simulink model "gm_parallel_lht"  (R2019b)
settings: Solver=FixedStepDiscrete  StartTime=0.0  StopTime=inf  RelTol=1e-3
undefined symbols (not defined in the file or in its folder): bt, height, width
libraries: hdlsllib x190, simulink x13, hdlmdlgenlib x7, dspsrcs4 x1
(part 2 of 18)

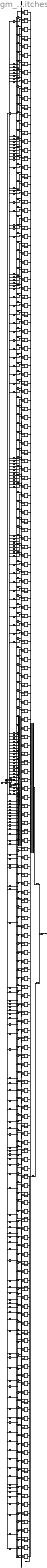
== system gm_parallel_lht/Parallel LHT/Parallel LHT Accumulator/Accumulator with Switches ==
  hough_address : Inport  OutDataTypeStr=fixdt(0, 11, 0)  PortDimensions=[1 180]  SampleTime=6.66666666666667e-09
  edge : Inport  Port=2  OutDataTypeStr=boolean  PortDimensions=1  SampleTime=6.66666666666667e-09
  mode : Inport  Port=3  OutDataTypeStr=boolean  PortDimensions=1  SampleTime=6.66666666666667e-09
  read_address : Inport  Port=4  OutDataTypeStr=uint16  PortDimensions=1  SampleTime=6.66666666666667e-09
  clear : Inport  Port=5  OutDataTypeStr=boolean  PortDimensions=1  SampleTime=6.66666666666667e-09
  theta_index : Inport  Port=6  OutDataTypeStr=uint16  PortDimensions=1  SampleTime=6.66666666666667e-09
  Accumulator_instance1 : Subsystem
  Accumulator_instance10 : Subsystem
  Accumulator_instance100 : Subsystem
  Accumulator_instance101 : Subsystem
  Accumulator_instance102 : Subsystem
  Accumulator_instance103 : Subsystem
  Accumulator_instance104 : Subsystem
  Accumulator_instance105 : Subsystem
  Accumulator_instance106 : Subsystem
  Accumulator_instance107 : Subsystem
  Accumulator_instance108 : Subsystem
  Accumulator_instance109 : Subsystem
  Accumulator_instance11 : Subsystem
  Accumulator_instance110 : Subsystem
  Accumulator_instance111 : Subsystem
  Accumulator_instance112 : Subsystem
  Accumulator_instance113 : Subsystem
  Accumulator_instance114 : Subsystem
  Accumulator_instance115 : Subsystem
  Accumulator_instance116 : Subsystem
  Accumulator_instance117 : Subsystem
  Accumulator_instance118 : Subsystem
  Accumulator_instance119 : Subsystem
  Accumulator_instance12 : Subsystem
  Accumulator_instance120 : Subsystem
  Accumulator_instance121 : Subsystem
  Accumulator_instance122 : Subsystem
  Accumulator_instance123 : Subsystem
  Accumulator_instance124 : Subsystem
  Accumulator_instance125 : Subsystem
  Accumulator_instance126 : Subsystem
  Accumulator_instance127 : Subsystem
  Accumulator_instance128 : Subsystem
  Accumulator_instance129 : Subsystem
  Accumulator_instance13 : Subsystem
  Accumulator_instance130 : Subsystem
  Accumulator_instance131 : Subsystem
  Accumulator_instance132 : Subsystem
  Accumulator_instance133 : Subsystem
  Accumulator_instance134 : Subsystem
  Accumulator_instance135 : Subsystem
  Accumulator_instance136 : Subsystem
  Accumulator_instance137 : Subsystem
  Accumulator_instance138 : Subsystem
  Accumulator_instance139 : Subsystem
  Accumulator_instance14 : Subsystem
  Accumulator_instance140 : Subsystem
  Accumulator_instance141 : Subsystem
  Accumulator_instance142 : Subsystem
  Accumulator_instance143 : Subsystem
  Accumulator_instance144 : Subsystem
  Accumulator_instance145 : Subsystem
  Accumulator_instance146 : Subsystem
  Accumulator_instance147 : Subsystem
  Accumulator_instance148 : Subsystem
  Accumulator_instance149 : Subsystem
  Accumulator_instance15 : Subsystem
  Accumulator_instance150 : Subsystem
  Accumulator_instance151 : Subsystem
  Accumulator_instance152 : Subsystem
  Accumulator_instance153 : Subsystem
  Accumulator_instance154 : Subsystem
  Accumulator_instance155 : Subsystem
  Accumulator_instance156 : Subsystem
  Accumulator_instance157 : Subsystem
  Accumulator_instance158 : Subsystem
  Accumulator_instance159 : Subsystem
  Accumulator_instance16 : Subsystem
  Accumulator_instance160 : Subsystem
  Accumulator_instance161 : Subsystem
  Accumulator_instance162 : Subsystem
  Accumulator_instance163 : Subsystem
  Accumulator_instance164 : Subsystem
  Accumulator_instance165 : Subsystem
  Accumulator_instance166 : Subsystem
  Accumulator_instance167 : Subsystem
  Accumulator_instance168 : Subsystem
  Accumulator_instance169 : Subsystem
  Accumulator_instance17 : Subsystem
  Accumulator_instance170 : Subsystem
  Accumulator_instance171 : Subsystem
  Accumulator_instance172 : Subsystem
  Accumulator_instance173 : Subsystem
  Accumulator_instance174 : Subsystem
  Accumulator_instance175 : Subsystem
  Accumulator_instance176 : Subsystem
  Accumulator_instance177 : Subsystem
  Accumulator_instance178 : Subsystem
  Accumulator_instance179 : Subsystem
  Accumulator_instance18 : Subsystem
  Accumulator_instance180 : Subsystem
  Accumulator_instance19 : Subsystem
  Accumulator_instance2 : Subsystem
  Accumulator_instance20 : Subsystem
  Accumulator_instance21 : Subsystem
  Accumulator_instance22 : Subsystem
  Accumulator_instance23 : Subsystem
  Accumulator_instance24 : Subsystem
  Accumulator_instance25 : Subsystem
  Accumulator_instance26 : Subsystem
  Accumulator_instance27 : Subsystem
  Accumulator_instance28 : Subsystem
  Accumulator_instance29 : Subsystem
  Accumulator_instance3 : Subsystem
  Accumulator_instance30 : Subsystem
  Accumulator_instance31 : Subsystem
  Accumulator_instance32 : Subsystem
  Accumulator_instance33 : Subsystem
  Accumulator_instance34 : Subsystem
  Accumulator_instance35 : Subsystem
  Accumulator_instance36 : Subsystem
  Accumulator_instance37 : Subsystem
  Accumulator_instance38 : Subsystem
  Accumulator_instance39 : Subsystem
  Accumulator_instance4 : Subsystem
  Accumulator_instance40 : Subsystem
  Accumulator_instance41 : Subsystem
  Accumulator_instance42 : Subsystem
  Accumulator_instance43 : Subsystem
  Accumulator_instance44 : Subsystem
  Accumulator_instance45 : Subsystem
  Accumulator_instance46 : Subsystem
  Accumulator_instance47 : Subsystem
  Accumulator_instance48 : Subsystem
  Accumulator_instance49 : Subsystem
  Accumulator_instance5 : Subsystem
  Accumulator_instance50 : Subsystem
  Accumulator_instance51 : Subsystem
  Accumulator_instance52 : Subsystem
  Accumulator_instance53 : Subsystem
  Accumulator_instance54 : Subsystem
  Accumulator_instance55 : Subsystem
  Accumulator_instance56 : Subsystem
  Accumulator_instance57 : Subsystem
  Accumulator_instance58 : Subsystem
  Accumulator_instance59 : Subsystem
  Accumulator_instance6 : Subsystem
  Accumulator_instance60 : Subsystem
  Accumulator_instance61 : Subsystem
  Accumulator_instance62 : Subsystem
  Accumulator_instance63 : Subsystem
  Accumulator_instance64 : Subsystem
  Accumulator_instance65 : Subsystem
  Accumulator_instance66 : Subsystem
  Accumulator_instance67 : Subsystem
  Accumulator_instance68 : Subsystem
  Accumulator_instance69 : Subsystem
  Accumulator_instance7 : Subsystem
  Accumulator_instance70 : Subsystem
  Accumulator_instance71 : Subsystem
  Accumulator_instance72 : Subsystem
  Accumulator_instance73 : Subsystem
  Accumulator_instance74 : Subsystem
  Accumulator_instance75 : Subsystem
  Accumulator_instance76 : Subsystem
  Accumulator_instance77 : Subsystem
  Accumulator_instance78 : Subsystem
  Accumulator_instance79 : Subsystem
  Accumulator_instance8 : Subsystem
  Accumulator_instance80 : Subsystem
  Accumulator_instance81 : Subsystem
  Accumulator_instance82 : Subsystem
  Accumulator_instance83 : Subsystem
  Accumulator_instance84 : Subsystem
  Accumulator_instance85 : Subsystem
  Accumulator_instance86 : Subsystem
  Accumulator_instance87 : Subsystem
  Accumulator_instance88 : Subsystem
  Accumulator_instance89 : Subsystem
  Accumulator_instance9 : Subsystem
  Accumulator_instance90 : Subsystem
  Accumulator_instance91 : Subsystem
  Accumulator_instance92 : Subsystem
  Accumulator_instance93 : Subsystem
  Accumulator_instance94 : Subsystem
  Accumulator_instance95 : Subsystem
  Accumulator_instance96 : Subsystem
  Accumulator_instance97 : Subsystem
  Accumulator_instance98 : Subsystem
  Accumulator_instance99 : Subsystem
  Data Type Conversion : DataTypeConversion  OutDataTypeStr=fixdt(0, 11, 0)  SampleTime=6.66666666666667e-09
  Delay : Delay  DelayLength=double(1)  InitialCondition=0  SampleTime=6.66666666666667e-09
  Multiport Switch1 : MultiPortSwitch  DataPortOrder=Zero-based contiguous  Inputs=2  DiagnosticForDefault=None  zeroidx=on  SampleTime=6.66666666666667e-09
  Selector : Selector  NumberOfDimensions=2  IndexMode=Zero-based  SampleTime=6.66666666666667e-09  IndexOptions=Index vector (dialog),Index vector (port)  Indices=double(0),double(0)  OutputSizes=double(1),double(1)
  Switch : Switch  Criteria=u2 > Threshold  Threshold=double(0)  OutDataTypeStr=fixdt(0, 11, 0)  SampleTime=6.66666666666667e-09
  delayMatch{,1..362} (363 alike) : Delay  DelayLength=double(2)  InitialCondition=0  SampleTime=6.66666666666667e-09
  t : Demux  Outputs=180
  t1 : Concatenate  NumInputs=180
  t2 : Reshape  OutputDimensionality=Row vector (2-D)
  hps : Outport
  wires:
  delayMatch/1 -> Switch/2
  t2/1 -> Selector/1
  delayMatch1/1 -> Switch/3
  delayMatch362/1 -> Selector/2
  delayMatch3/1 -> Accumulator_instance1/3(edge)
  Selector/1 -> hps/1
  Switch/1 -> t/1
  t/1 -> Accumulator_instance1/2(address)
  t/2 -> Accumulator_instance2/2(address)
  t/3 -> Accumulator_instance3/2(address)
  t/4 -> Accumulator_instance4/2(address)
  t/5 -> Accumulator_instance5/2(address)
  t/6 -> Accumulator_instance6/2(address)
  t/7 -> Accumulator_instance7/2(address)
  t/8 -> Accumulator_instance8/2(address)
  t/9 -> Accumulator_instance9/2(address)
  t/10 -> Accumulator_instance10/2(address)
  t/11 -> Accumulator_instance11/2(address)
  t/12 -> Accumulator_instance12/2(address)
  t/13 -> Accumulator_instance13/2(address)
  t/14 -> Accumulator_instance14/2(address)
  t/15 -> Accumulator_instance15/2(address)
  t/16 -> Accumulator_instance16/2(address)
  t/17 -> Accumulator_instance17/2(address)
  t/18 -> Accumulator_instance18/2(address)
  t/19 -> Accumulator_instance19/2(address)
  t/20 -> Accumulator_instance20/2(address)
  t/21 -> Accumulator_instance21/2(address)
  t/22 -> Accumulator_instance22/2(address)
  t/23 -> Accumulator_instance23/2(address)
  t/24 -> Accumulator_instance24/2(address)
  t/25 -> Accumulator_instance25/2(address)
  t/26 -> Accumulator_instance26/2(address)
  t/27 -> Accumulator_instance27/2(address)
  t/28 -> Accumulator_instance28/2(address)
  t/29 -> Accumulator_instance29/2(address)
  t/30 -> Accumulator_instance30/2(address)
  t/31 -> Accumulator_instance31/2(address)
  t/32 -> Accumulator_instance32/2(address)
  t/33 -> Accumulator_instance33/2(address)
  t/34 -> Accumulator_instance34/2(address)
  t/35 -> Accumulator_instance35/2(address)
  t/36 -> Accumulator_instance36/2(address)
  t/37 -> Accumulator_instance37/2(address)
  t/38 -> Accumulator_instance38/2(address)
  t/39 -> Accumulator_instance39/2(address)
  t/40 -> Accumulator_instance40/2(address)
  t/41 -> Accumulator_instance41/2(address)
  t/42 -> Accumulator_instance42/2(address)
  t/43 -> Accumulator_instance43/2(address)
  t/44 -> Accumulator_instance44/2(address)
  t/45 -> Accumulator_instance45/2(address)
  t/46 -> Accumulator_instance46/2(address)
  t/47 -> Accumulator_instance47/2(address)
  t/48 -> Accumulator_instance48/2(address)
  t/49 -> Accumulator_instance49/2(address)
  t/50 -> Accumulator_instance50/2(address)
  t/51 -> Accumulator_instance51/2(address)
  t/52 -> Accumulator_instance52/2(address)
  t/53 -> Accumulator_instance53/2(address)
  t/54 -> Accumulator_instance54/2(address)
  t/55 -> Accumulator_instance55/2(address)
  t/56 -> Accumulator_instance56/2(address)
  t/57 -> Accumulator_instance57/2(address)
  t/58 -> Accumulator_instance58/2(address)
  t/59 -> Accumulator_instance59/2(address)
  t/60 -> Accumulator_instance60/2(address)
  t/61 -> Accumulator_instance61/2(address)
  t/62 -> Accumulator_instance62/2(address)
  t/63 -> Accumulator_instance63/2(address)
  t/64 -> Accumulator_instance64/2(address)
  t/65 -> Accumulator_instance65/2(address)
  t/66 -> Accumulator_instance66/2(address)
  t/67 -> Accumulator_instance67/2(address)
  t/68 -> Accumulator_instance68/2(address)
  t/69 -> Accumulator_instance69/2(address)
  t/70 -> Accumulator_instance70/2(address)
  t/71 -> Accumulator_instance71/2(address)
  t/72 -> Accumulator_instance72/2(address)
  t/73 -> Accumulator_instance73/2(address)
  t/74 -> Accumulator_instance74/2(address)
  t/75 -> Accumulator_instance75/2(address)
  t/76 -> Accumulator_instance76/2(address)
  t/77 -> Accumulator_instance77/2(address)
  t/78 -> Accumulator_instance78/2(address)
  t/79 -> Accumulator_instance79/2(address)
  t/80 -> Accumulator_instance80/2(address)
  t/81 -> Accumulator_instance81/2(address)
  t/82 -> Accumulator_instance82/2(address)
  t/83 -> Accumulator_instance83/2(address)
  t/84 -> Accumulator_instance84/2(address)
  t/85 -> Accumulator_instance85/2(address)
  t/86 -> Accumulator_instance86/2(address)
  t/87 -> Accumulator_instance87/2(address)
  t/88 -> Accumulator_instance88/2(address)
  t/89 -> Accumulator_instance89/2(address)
  t/90 -> Accumulator_instance90/2(address)
  t/91 -> Accumulator_instance91/2(address)
  t/92 -> Accumulator_instance92/2(address)
  t/93 -> Accumulator_instance93/2(address)
  t/94 -> Accumulator_instance94/2(address)
  t/95 -> Accumulator_instance95/2(address)
  t/96 -> Accumulator_instance96/2(address)
  t/97 -> Accumulator_instance97/2(address)
  t/98 -> Accumulator_instance98/2(address)
  t/99 -> Accumulator_instance99/2(address)
  t/100 -> Accumulator_instance100/2(address)
  t/101 -> Accumulator_instance101/2(address)
  t/102 -> Accumulator_instance102/2(address)
  t/103 -> Accumulator_instance103/2(address)
  t/104 -> Accumulator_instance104/2(address)
  t/105 -> Accumulator_instance105/2(address)
  t/106 -> Accumulator_instance106/2(address)
  t/107 -> Accumulator_instance107/2(address)
  t/108 -> Accumulator_instance108/2(address)
  t/109 -> Accumulator_instance109/2(address)
  t/110 -> Accumulator_instance110/2(address)
  t/111 -> Accumulator_instance111/2(address)
  t/112 -> Accumulator_instance112/2(address)
  t/113 -> Accumulator_instance113/2(address)
  t/114 -> Accumulator_instance114/2(address)
  t/115 -> Accumulator_instance115/2(address)
  t/116 -> Accumulator_instance116/2(address)
  t/117 -> Accumulator_instance117/2(address)
  t/118 -> Accumulator_instance118/2(address)
  t/119 -> Accumulator_instance119/2(address)
  t/120 -> Accumulator_instance120/2(address)
  t/121 -> Accumulator_instance121/2(address)
  t/122 -> Accumulator_instance122/2(address)
  t/123 -> Accumulator_instance123/2(address)
  t/124 -> Accumulator_instance124/2(address)
  t/125 -> Accumulator_instance125/2(address)
  t/126 -> Accumulator_instance126/2(address)
  t/127 -> Accumulator_instance127/2(address)
  t/128 -> Accumulator_instance128/2(address)
  t/129 -> Accumulator_instance129/2(address)
  t/130 -> Accumulator_instance130/2(address)
  t/131 -> Accumulator_instance131/2(address)
  t/132 -> Accumulator_instance132/2(address)
  t/133 -> Accumulator_instance133/2(address)
  t/134 -> Accumulator_instance134/2(address)
  t/135 -> Accumulator_instance135/2(address)
  t/136 -> Accumulator_instance136/2(address)
  t/137 -> Accumulator_instance137/2(address)
  t/138 -> Accumulator_instance138/2(address)
  t/139 -> Accumulator_instance139/2(address)
  t/140 -> Accumulator_instance140/2(address)
  t/141 -> Accumulator_instance141/2(address)
  t/142 -> Accumulator_instance142/2(address)
  t/143 -> Accumulator_instance143/2(address)
  t/144 -> Accumulator_instance144/2(address)
  t/145 -> Accumulator_instance145/2(address)
  t/146 -> Accumulator_instance146/2(address)
  t/147 -> Accumulator_instance147/2(address)
  t/148 -> Accumulator_instance148/2(address)
  t/149 -> Accumulator_instance149/2(address)
  t/150 -> Accumulator_instance150/2(address)
  t/151 -> Accumulator_instance151/2(address)
  t/152 -> Accumulator_instance152/2(address)
  t/153 -> Accumulator_instance153/2(address)
  t/154 -> Accumulator_instance154/2(address)
  t/155 -> Accumulator_instance155/2(address)
  t/156 -> Accumulator_instance156/2(address)
  t/157 -> Accumulator_instance157/2(address)
  t/158 -> Accumulator_instance158/2(address)
  t/159 -> Accumulator_instance159/2(address)
  t/160 -> Accumulator_instance160/2(address)
  t/161 -> Accumulator_instance161/2(address)
  t/162 -> Accumulator_instance162/2(address)
  t/163 -> Accumulator_instance163/2(address)
  t/164 -> Accumulator_instance164/2(address)
  t/165 -> Accumulator_instance165/2(address)
  t/166 -> Accumulator_instance166/2(address)
  t/167 -> Accumulator_instance167/2(address)
  t/168 -> Accumulator_instance168/2(address)
  t/169 -> Accumulator_instance169/2(address)
  t/170 -> Accumulator_instance170/2(address)
  t/171 -> Accumulator_instance171/2(address)
  t/172 -> Accumulator_instance172/2(address)
  t/173 -> Accumulator_instance173/2(address)
  t/174 -> Accumulator_instance174/2(address)
  t/175 -> Accumulator_instance175/2(address)
  t/176 -> Accumulator_instance176/2(address)
  t/177 -> Accumulator_instance177/2(address)
  t/178 -> Accumulator_instance178/2(address)
  t/179 -> Accumulator_instance179/2(address)
  t/180 -> Accumulator_instance180/2(address)
  t1/1 -> t2/1
  Accumulator_instance1/1(hps) -> t1/1
  Accumulator_instance2/1(hps) -> t1/2
  Accumulator_instance3/1(hps) -> t1/3
  Accumulator_instance4/1(hps) -> t1/4
  Accumulator_instance5/1(hps) -> t1/5
  Accumulator_instance6/1(hps) -> t1/6
  Accumulator_instance7/1(hps) -> t1/7
  Accumulator_instance8/1(hps) -> t1/8
  Accumulator_instance9/1(hps) -> t1/9
  Accumulator_instance10/1(hps) -> t1/10
  Accumulator_instance11/1(hps) -> t1/11
  Accumulator_instance12/1(hps) -> t1/12
  Accumulator_instance13/1(hps) -> t1/13
  Accumulator_instance14/1(hps) -> t1/14
  Accumulator_instance15/1(hps) -> t1/15
  Accumulator_instance16/1(hps) -> t1/16
  Accumulator_instance17/1(hps) -> t1/17
  Accumulator_instance18/1(hps) -> t1/18
  Accumulator_instance19/1(hps) -> t1/19
  Accumulator_instance20/1(hps) -> t1/20
  Accumulator_instance21/1(hps) -> t1/21
  Accumulator_instance22/1(hps) -> t1/22
  Accumulator_instance23/1(hps) -> t1/23
  Accumulator_instance24/1(hps) -> t1/24
  Accumulator_instance25/1(hps) -> t1/25
  Accumulator_instance26/1(hps) -> t1/26
  Accumulator_instance27/1(hps) -> t1/27
  Accumulator_instance28/1(hps) -> t1/28
  Accumulator_instance29/1(hps) -> t1/29
  Accumulator_instance30/1(hps) -> t1/30
  Accumulator_instance31/1(hps) -> t1/31
  Accumulator_instance32/1(hps) -> t1/32
  Accumulator_instance33/1(hps) -> t1/33
  Accumulator_instance34/1(hps) -> t1/34
  Accumulator_instance35/1(hps) -> t1/35
  Accumulator_instance36/1(hps) -> t1/36
  Accumulator_instance37/1(hps) -> t1/37
  Accumulator_instance38/1(hps) -> t1/38
  Accumulator_instance39/1(hps) -> t1/39
  Accumulator_instance40/1(hps) -> t1/40
  Accumulator_instance41/1(hps) -> t1/41
  Accumulator_instance42/1(hps) -> t1/42
  Accumulator_instance43/1(hps) -> t1/43
  Accumulator_instance44/1(hps) -> t1/44
  Accumulator_instance45/1(hps) -> t1/45
  Accumulator_instance46/1(hps) -> t1/46
  Accumulator_instance47/1(hps) -> t1/47
  Accumulator_instance48/1(hps) -> t1/48
  Accumulator_instance49/1(hps) -> t1/49
  Accumulator_instance50/1(hps) -> t1/50
  Accumulator_instance51/1(hps) -> t1/51
  Accumulator_instance52/1(hps) -> t1/52
  Accumulator_instance53/1(hps) -> t1/53
  Accumulator_instance54/1(hps) -> t1/54
  Accumulator_instance55/1(hps) -> t1/55
  Accumulator_instance56/1(hps) -> t1/56
  Accumulator_instance57/1(hps) -> t1/57
  Accumulator_instance58/1(hps) -> t1/58
  Accumulator_instance59/1(hps) -> t1/59
  Accumulator_instance60/1(hps) -> t1/60
  Accumulator_instance61/1(hps) -> t1/61
  Accumulator_instance62/1(hps) -> t1/62
  Accumulator_instance63/1(hps) -> t1/63
  Accumulator_instance64/1(hps) -> t1/64
  Accumulator_instance65/1(hps) -> t1/65
  Accumulator_instance66/1(hps) -> t1/66
  Accumulator_instance67/1(hps) -> t1/67
  Accumulator_instance68/1(hps) -> t1/68
  Accumulator_instance69/1(hps) -> t1/69
  Accumulator_instance70/1(hps) -> t1/70
  Accumulator_instance71/1(hps) -> t1/71
  Accumulator_instance72/1(hps) -> t1/72
  Accumulator_instance73/1(hps) -> t1/73
  Accumulator_instance74/1(hps) -> t1/74
  Accumulator_instance75/1(hps) -> t1/75
  Accumulator_instance76/1(hps) -> t1/76
  Accumulator_instance77/1(hps) -> t1/77
  Accumulator_instance78/1(hps) -> t1/78
  Accumulator_instance79/1(hps) -> t1/79
  Accumulator_instance80/1(hps) -> t1/80
  Accumulator_instance81/1(hps) -> t1/81
  Accumulator_instance82/1(hps) -> t1/82
  Accumulator_instance83/1(hps) -> t1/83
  Accumulator_instance84/1(hps) -> t1/84
  Accumulator_instance85/1(hps) -> t1/85
  Accumulator_instance86/1(hps) -> t1/86
  Accumulator_instance87/1(hps) -> t1/87
  Accumulator_instance88/1(hps) -> t1/88
  Accumulator_instance89/1(hps) -> t1/89
  Accumulator_instance90/1(hps) -> t1/90
  Accumulator_instance91/1(hps) -> t1/91
  Accumulator_instance92/1(hps) -> t1/92
  Accumulator_instance93/1(hps) -> t1/93
  Accumulator_instance94/1(hps) -> t1/94
  Accumulator_instance95/1(hps) -> t1/95
  Accumulator_instance96/1(hps) -> t1/96
  Accumulator_instance97/1(hps) -> t1/97
  Accumulator_instance98/1(hps) -> t1/98
  Accumulator_instance99/1(hps) -> t1/99
  Accumulator_instance100/1(hps) -> t1/100
  Accumulator_instance101/1(hps) -> t1/101
  Accumulator_instance102/1(hps) -> t1/102
  Accumulator_instance103/1(hps) -> t1/103
  Accumulator_instance104/1(hps) -> t1/104
  Accumulator_instance105/1(hps) -> t1/105
  Accumulator_instance106/1(hps) -> t1/106
  Accumulator_instance107/1(hps) -> t1/107
  Accumulator_instance108/1(hps) -> t1/108
  Accumulator_instance109/1(hps) -> t1/109
  Accumulator_instance110/1(hps) -> t1/110
  Accumulator_instance111/1(hps) -> t1/111
  Accumulator_instance112/1(hps) -> t1/112
  Accumulator_instance113/1(hps) -> t1/113
  Accumulator_instance114/1(hps) -> t1/114
  Accumulator_instance115/1(hps) -> t1/115
  Accumulator_instance116/1(hps) -> t1/116
  Accumulator_instance117/1(hps) -> t1/117
  Accumulator_instance118/1(hps) -> t1/118
  Accumulator_instance119/1(hps) -> t1/119
  Accumulator_instance120/1(hps) -> t1/120
  Accumulator_instance121/1(hps) -> t1/121
  Accumulator_instance122/1(hps) -> t1/122
  Accumulator_instance123/1(hps) -> t1/123
  Accumulator_instance124/1(hps) -> t1/124
  Accumulator_instance125/1(hps) -> t1/125
  Accumulator_instance126/1(hps) -> t1/126
  Accumulator_instance127/1(hps) -> t1/127
  Accumulator_instance128/1(hps) -> t1/128
  Accumulator_instance129/1(hps) -> t1/129
  Accumulator_instance130/1(hps) -> t1/130
  Accumulator_instance131/1(hps) -> t1/131
  Accumulator_instance132/1(hps) -> t1/132
  Accumulator_instance133/1(hps) -> t1/133
  Accumulator_instance134/1(hps) -> t1/134
  Accumulator_instance135/1(hps) -> t1/135
  Accumulator_instance136/1(hps) -> t1/136
  Accumulator_instance137/1(hps) -> t1/137
  Accumulator_instance138/1(hps) -> t1/138
  Accumulator_instance139/1(hps) -> t1/139
  Accumulator_instance140/1(hps) -> t1/140
  Accumulator_instance141/1(hps) -> t1/141
  Accumulator_instance142/1(hps) -> t1/142
  Accumulator_instance143/1(hps) -> t1/143
  Accumulator_instance144/1(hps) -> t1/144
  Accumulator_instance145/1(hps) -> t1/145
  Accumulator_instance146/1(hps) -> t1/146
  Accumulator_instance147/1(hps) -> t1/147
  Accumulator_instance148/1(hps) -> t1/148
  Accumulator_instance149/1(hps) -> t1/149
  Accumulator_instance150/1(hps) -> t1/150
  Accumulator_instance151/1(hps) -> t1/151
  Accumulator_instance152/1(hps) -> t1/152
  Accumulator_instance153/1(hps) -> t1/153
  Accumulator_instance154/1(hps) -> t1/154
  Accumulator_instance155/1(hps) -> t1/155
  Accumulator_instance156/1(hps) -> t1/156
  Accumulator_instance157/1(hps) -> t1/157
  Accumulator_instance158/1(hps) -> t1/158
  Accumulator_instance159/1(hps) -> t1/159
  Accumulator_instance160/1(hps) -> t1/160
  Accumulator_instance161/1(hps) -> t1/161
  Accumulator_instance162/1(hps) -> t1/162
  Accumulator_instance163/1(hps) -> t1/163
  Accumulator_instance164/1(hps) -> t1/164
  Accumulator_instance165/1(hps) -> t1/165
  Accumulator_instance166/1(hps) -> t1/166
  Accumulator_instance167/1(hps) -> t1/167
  Accumulator_instance168/1(hps) -> t1/168
  Accumulator_instance169/1(hps) -> t1/169
  Accumulator_instance170/1(hps) -> t1/170
  Accumulator_instance171/1(hps) -> t1/171
  Accumulator_instance172/1(hps) -> t1/172
  Accumulator_instance173/1(hps) -> t1/173
  Accumulator_instance174/1(hps) -> t1/174
  Accumulator_instance175/1(hps) -> t1/175
  Accumulator_instance176/1(hps) -> t1/176
  Accumulator_instance177/1(hps) -> t1/177
  Accumulator_instance178/1(hps) -> t1/178
  Accumulator_instance179/1(hps) -> t1/179
  Accumulator_instance180/1(hps) -> t1/180
  hough_address/1 -> Switch/1
  edge/1 -> Multiport Switch1/3
  mode/1 -> delayMatch360/1, delayMatch358/1, delayMatch356/1, delayMatch354/1, delayMatch352/1, delayMatch350/1, delayMatch348/1, delayMatch346/1, delayMatch344/1, delayMatch342/1, delayMatch340/1, delayMatch338/1, delayMatch336/1, delayMatch334/1, delayMatch332/1, delayMatch330/1, delayMatch328/1, delayMatch326/1, delayMatch324/1, delayMatch322/1, delayMatch320/1, delayMatch318/1, delayMatch316/1, delayMatch314/1, delayMatch312/1, delayMatch310/1, delayMatch308/1, delayMatch306/1, delayMatch304/1, delayMatch302/1, delayMatch300/1, delayMatch298/1, delayMatch296/1, delayMatch294/1, delayMatch292/1, delayMatch290/1, delayMatch288/1, delayMatch286/1, delayMatch284/1, delayMatch282/1, delayMatch280/1, delayMatch278/1, delayMatch276/1, delayMatch274/1, delayMatch272/1, delayMatch270/1, delayMatch268/1, delayMatch266/1, delayMatch264/1, delayMatch262/1, delayMatch260/1, delayMatch258/1, delayMatch256/1, delayMatch254/1, delayMatch252/1, delayMatch250/1, delayMatch248/1, delayMatch246/1, delayMatch244/1, delayMatch242/1, delayMatch240/1, delayMatch238/1, delayMatch236/1, delayMatch234/1, delayMatch232/1, delayMatch230/1, delayMatch228/1, delayMatch226/1, delayMatch224/1, delayMatch222/1, delayMatch220/1, delayMatch218/1, delayMatch216/1, delayMatch214/1, delayMatch212/1, delayMatch210/1, delayMatch208/1, delayMatch206/1, delayMatch204/1, delayMatch202/1, delayMatch200/1, delayMatch198/1, delayMatch196/1, delayMatch194/1, delayMatch192/1, delayMatch190/1, delayMatch188/1, delayMatch186/1, delayMatch184/1, delayMatch182/1, delayMatch180/1, delayMatch178/1, delayMatch176/1, delayMatch174/1, delayMatch172/1, delayMatch170/1, delayMatch168/1, delayMatch166/1, delayMatch164/1, delayMatch162/1, delayMatch160/1, delayMatch158/1, delayMatch156/1, delayMatch154/1, delayMatch152/1, delayMatch150/1, delayMatch148/1, delayMatch146/1, delayMatch144/1, delayMatch142/1, delayMatch140/1, delayMatch138/1, delayMatch136/1, delayMatch134/1, delayMatch132/1, delayMatch130/1, delayMatch128/1, delayMatch126/1, delayMatch124/1, delayMatch122/1, delayMatch120/1, delayMatch118/1, delayMatch116/1, delayMatch114/1, delayMatch112/1, delayMatch110/1, delayMatch108/1, delayMatch106/1, delayMatch104/1, delayMatch102/1, delayMatch100/1, delayMatch98/1, delayMatch96/1, delayMatch94/1, delayMatch92/1, delayMatch90/1, delayMatch88/1, delayMatch86/1, delayMatch84/1, delayMatch82/1, delayMatch80/1, delayMatch78/1, delayMatch76/1, delayMatch74/1, delayMatch72/1, delayMatch70/1, delayMatch68/1, delayMatch66/1, delayMatch64/1, delayMatch62/1, delayMatch60/1, delayMatch58/1, delayMatch56/1, delayMatch54/1, delayMatch52/1, delayMatch50/1, delayMatch48/1, delayMatch46/1, delayMatch44/1, delayMatch42/1, delayMatch40/1, delayMatch38/1, delayMatch36/1, delayMatch34/1, delayMatch32/1, delayMatch30/1, delayMatch28/1, delayMatch26/1, delayMatch24/1, delayMatch22/1, delayMatch20/1, delayMatch18/1, delayMatch16/1, delayMatch14/1, delayMatch12/1, delayMatch10/1, delayMatch8/1, delayMatch6/1, delayMatch4/1, delayMatch2/1, delayMatch/1, Multiport Switch1/1
  read_address/1 -> Data Type Conversion/1
  clear/1 -> Multiport Switch1/2
  theta_index/1 -> Delay/1
  delayMatch2/1 -> Accumulator_instance1/1(mode)
  Data Type Conversion/1 -> delayMatch1/1
  delayMatch4/1 -> Accumulator_instance2/1(mode)
  delayMatch5/1 -> Accumulator_instance2/3(edge)
  delayMatch6/1 -> Accumulator_instance3/1(mode)
  delayMatch7/1 -> Accumulator_instance3/3(edge)
  delayMatch8/1 -> Accumulator_instance4/1(mode)
  delayMatch9/1 -> Accumulator_instance4/3(edge)
  delayMatch10/1 -> Accumulator_instance5/1(mode)
  delayMatch11/1 -> Accumulator_instance5/3(edge)
  delayMatch12/1 -> Accumulator_instance6/1(mode)
  delayMatch13/1 -> Accumulator_instance6/3(edge)
  delayMatch14/1 -> Accumulator_instance7/1(mode)
  delayMatch15/1 -> Accumulator_instance7/3(edge)
  delayMatch16/1 -> Accumulator_instance8/1(mode)
  delayMatch17/1 -> Accumulator_instance8/3(edge)
  delayMatch18/1 -> Accumulator_instance9/1(mode)
  delayMatch19/1 -> Accumulator_instance9/3(edge)
  delayMatch20/1 -> Accumulator_instance10/1(mode)
  delayMatch21/1 -> Accumulator_instance10/3(edge)
  delayMatch22/1 -> Accumulator_instance11/1(mode)
  delayMatch23/1 -> Accumulator_instance11/3(edge)
  delayMatch24/1 -> Accumulator_instance12/1(mode)
  delayMatch25/1 -> Accumulator_instance12/3(edge)
  delayMatch26/1 -> Accumulator_instance13/1(mode)
  delayMatch27/1 -> Accumulator_instance13/3(edge)
  delayMatch28/1 -> Accumulator_instance14/1(mode)
  delayMatch29/1 -> Accumulator_instance14/3(edge)
  delayMatch30/1 -> Accumulator_instance15/1(mode)
  delayMatch31/1 -> Accumulator_instance15/3(edge)
  delayMatch32/1 -> Accumulator_instance16/1(mode)
  delayMatch33/1 -> Accumulator_instance16/3(edge)
  delayMatch34/1 -> Accumulator_instance17/1(mode)
  delayMatch35/1 -> Accumulator_instance17/3(edge)
  delayMatch36/1 -> Accumulator_instance18/1(mode)
  delayMatch37/1 -> Accumulator_instance18/3(edge)
  delayMatch38/1 -> Accumulator_instance19/1(mode)
  delayMatch39/1 -> Accumulator_instance19/3(edge)
  delayMatch40/1 -> Accumulator_instance20/1(mode)
  delayMatch41/1 -> Accumulator_instance20/3(edge)
  delayMatch42/1 -> Accumulator_instance21/1(mode)
  delayMatch43/1 -> Accumulator_instance21/3(edge)
  delayMatch44/1 -> Accumulator_instance22/1(mode)
  delayMatch45/1 -> Accumulator_instance22/3(edge)
  delayMatch46/1 -> Accumulator_instance23/1(mode)
  delayMatch47/1 -> Accumulator_instance23/3(edge)
  delayMatch48/1 -> Accumulator_instance24/1(mode)
  delayMatch49/1 -> Accumulator_instance24/3(edge)
  delayMatch50/1 -> Accumulator_instance25/1(mode)
  delayMatch51/1 -> Accumulator_instance25/3(edge)
  delayMatch52/1 -> Accumulator_instance26/1(mode)
  delayMatch53/1 -> Accumulator_instance26/3(edge)
  delayMatch54/1 -> Accumulator_instance27/1(mode)
  delayMatch55/1 -> Accumulator_instance27/3(edge)
  delayMatch56/1 -> Accumulator_instance28/1(mode)
  delayMatch57/1 -> Accumulator_instance28/3(edge)
  delayMatch58/1 -> Accumulator_instance29/1(mode)
  delayMatch59/1 -> Accumulator_instance29/3(edge)
  delayMatch60/1 -> Accumulator_instance30/1(mode)
  delayMatch61/1 -> Accumulator_instance30/3(edge)
  delayMatch62/1 -> Accumulator_instance31/1(mode)
  delayMatch63/1 -> Accumulator_instance31/3(edge)
  delayMatch64/1 -> Accumulator_instance32/1(mode)
  delayMatch65/1 -> Accumulator_instance32/3(edge)
  delayMatch66/1 -> Accumulator_instance33/1(mode)
  delayMatch67/1 -> Accumulator_instance33/3(edge)
  delayMatch68/1 -> Accumulator_instance34/1(mode)
  delayMatch69/1 -> Accumulator_instance34/3(edge)
  delayMatch70/1 -> Accumulator_instance35/1(mode)
  delayMatch71/1 -> Accumulator_instance35/3(edge)
  delayMatch72/1 -> Accumulator_instance36/1(mode)
  delayMatch73/1 -> Accumulator_instance36/3(edge)
  delayMatch74/1 -> Accumulator_instance37/1(mode)
  delayMatch75/1 -> Accumulator_instance37/3(edge)
  delayMatch76/1 -> Accumulator_instance38/1(mode)
  delayMatch77/1 -> Accumulator_instance38/3(edge)
  delayMatch78/1 -> Accumulator_instance39/1(mode)
  delayMatch79/1 -> Accumulator_instance39/3(edge)
  delayMatch80/1 -> Accumulator_instance40/1(mode)
  delayMatch81/1 -> Accumulator_instance40/3(edge)
  delayMatch82/1 -> Accumulator_instance41/1(mode)
  delayMatch83/1 -> Accumulator_instance41/3(edge)
  delayMatch84/1 -> Accumulator_instance42/1(mode)
  delayMatch85/1 -> Accumulator_instance42/3(edge)
  delayMatch86/1 -> Accumulator_instance43/1(mode)
  delayMatch87/1 -> Accumulator_instance43/3(edge)
  delayMatch88/1 -> Accumulator_instance44/1(mode)
  delayMatch89/1 -> Accumulator_instance44/3(edge)
  delayMatch90/1 -> Accumulator_instance45/1(mode)
  delayMatch91/1 -> Accumulator_instance45/3(edge)
  delayMatch92/1 -> Accumulator_instance46/1(mode)
  delayMatch93/1 -> Accumulator_instance46/3(edge)
  delayMatch94/1 -> Accumulator_instance47/1(mode)
  delayMatch95/1 -> Accumulator_instance47/3(edge)
  delayMatch96/1 -> Accumulator_instance48/1(mode)
  delayMatch97/1 -> Accumulator_instance48/3(edge)
  delayMatch98/1 -> Accumulator_instance49/1(mode)
  delayMatch99/1 -> Accumulator_instance49/3(edge)
  delayMatch100/1 -> Accumulator_instance50/1(mode)
  delayMatch101/1 -> Accumulator_instance50/3(edge)
  delayMatch102/1 -> Accumulator_instance51/1(mode)
  delayMatch103/1 -> Accumulator_instance51/3(edge)
  delayMatch104/1 -> Accumulator_instance52/1(mode)
  delayMatch105/1 -> Accumulator_instance52/3(edge)
  delayMatch106/1 -> Accumulator_instance53/1(mode)
  delayMatch107/1 -> Accumulator_instance53/3(edge)
  delayMatch108/1 -> Accumulator_instance54/1(mode)
  delayMatch109/1 -> Accumulator_instance54/3(edge)
  delayMatch110/1 -> Accumulator_instance55/1(mode)
  delayMatch111/1 -> Accumulator_instance55/3(edge)
  delayMatch112/1 -> Accumulator_instance56/1(mode)
  delayMatch113/1 -> Accumulator_instance56/3(edge)
  delayMatch114/1 -> Accumulator_instance57/1(mode)
  delayMatch115/1 -> Accumulator_instance57/3(edge)
  delayMatch116/1 -> Accumulator_instance58/1(mode)
  delayMatch117/1 -> Accumulator_instance58/3(edge)
  delayMatch118/1 -> Accumulator_instance59/1(mode)
  delayMatch119/1 -> Accumulator_instance59/3(edge)
  delayMatch120/1 -> Accumulator_instance60/1(mode)
  delayMatch121/1 -> Accumulator_instance60/3(edge)
  delayMatch122/1 -> Accumulator_instance61/1(mode)
  delayMatch123/1 -> Accumulator_instance61/3(edge)
  delayMatch124/1 -> Accumulator_instance62/1(mode)
  delayMatch125/1 -> Accumulator_instance62/3(edge)
  delayMatch126/1 -> Accumulator_instance63/1(mode)
  delayMatch127/1 -> Accumulator_instance63/3(edge)
  delayMatch128/1 -> Accumulator_instance64/1(mode)
  delayMatch129/1 -> Accumulator_instance64/3(edge)
  delayMatch130/1 -> Accumulator_instance65/1(mode)
  delayMatch131/1 -> Accumulator_instance65/3(edge)
  delayMatch132/1 -> Accumulator_instance66/1(mode)
  delayMatch133/1 -> Accumulator_instance66/3(edge)
  delayMatch134/1 -> Accumulator_instance67/1(mode)
  delayMatch135/1 -> Accumulator_instance67/3(edge)
  delayMatch136/1 -> Accumulator_instance68/1(mode)
  delayMatch137/1 -> Accumulator_instance68/3(edge)
  delayMatch138/1 -> Accumulator_instance69/1(mode)
  delayMatch139/1 -> Accumulator_instance69/3(edge)
  delayMatch140/1 -> Accumulator_instance70/1(mode)
  delayMatch141/1 -> Accumulator_instance70/3(edge)
  delayMatch142/1 -> Accumulator_instance71/1(mode)
  delayMatch143/1 -> Accumulator_instance71/3(edge)
  delayMatch144/1 -> Accumulator_instance72/1(mode)
  delayMatch145/1 -> Accumulator_instance72/3(edge)
  delayMatch146/1 -> Accumulator_instance73/1(mode)
  delayMatch147/1 -> Accumulator_instance73/3(edge)
  delayMatch148/1 -> Accumulator_instance74/1(mode)
  delayMatch149/1 -> Accumulator_instance74/3(edge)
  delayMatch150/1 -> Accumulator_instance75/1(mode)
  delayMatch151/1 -> Accumulator_instance75/3(edge)
  delayMatch152/1 -> Accumulator_instance76/1(mode)
  delayMatch153/1 -> Accumulator_instance76/3(edge)
  delayMatch154/1 -> Accumulator_instance77/1(mode)
  delayMatch155/1 -> Accumulator_instance77/3(edge)
  delayMatch156/1 -> Accumulator_instance78/1(mode)
  delayMatch157/1 -> Accumulator_instance78/3(edge)
  delayMatch158/1 -> Accumulator_instance79/1(mode)
  delayMatch159/1 -> Accumulator_instance79/3(edge)
  delayMatch160/1 -> Accumulator_instance80/1(mode)
  delayMatch161/1 -> Accumulator_instance80/3(edge)
  delayMatch162/1 -> Accumulator_instance81/1(mode)
  delayMatch163/1 -> Accumulator_instance81/3(edge)
  delayMatch164/1 -> Accumulator_instance82/1(mode)
  delayMatch165/1 -> Accumulator_instance82/3(edge)
  delayMatch166/1 -> Accumulator_instance83/1(mode)
  delayMatch167/1 -> Accumulator_instance83/3(edge)
  delayMatch168/1 -> Accumulator_instance84/1(mode)
  delayMatch169/1 -> Accumulator_instance84/3(edge)
  delayMatch170/1 -> Accumulator_instance85/1(mode)
  delayMatch171/1 -> Accumulator_instance85/3(edge)
  delayMatch172/1 -> Accumulator_instance86/1(mode)
  delayMatch173/1 -> Accumulator_instance86/3(edge)
  delayMatch174/1 -> Accumulator_instance87/1(mode)
  delayMatch175/1 -> Accumulator_instance87/3(edge)
  delayMatch176/1 -> Accumulator_instance88/1(mode)
  delayMatch177/1 -> Accumulator_instance88/3(edge)
  delayMatch178/1 -> Accumulator_instance89/1(mode)
  delayMatch179/1 -> Accumulator_instance89/3(edge)
  delayMatch180/1 -> Accumulator_instance90/1(mode)
  delayMatch181/1 -> Accumulator_instance90/3(edge)
  delayMatch182/1 -> Accumulator_instance91/1(mode)
  delayMatch183/1 -> Accumulator_instance91/3(edge)
  delayMatch184/1 -> Accumulator_instance92/1(mode)
  delayMatch185/1 -> Accumulator_instance92/3(edge)
  delayMatch186/1 -> Accumulator_instance93/1(mode)
  delayMatch187/1 -> Accumulator_instance93/3(edge)
  delayMatch188/1 -> Accumulator_instance94/1(mode)
  delayMatch189/1 -> Accumulator_instance94/3(edge)
  delayMatch190/1 -> Accumulator_instance95/1(mode)
  delayMatch191/1 -> Accumulator_instance95/3(edge)
  delayMatch192/1 -> Accumulator_instance96/1(mode)
  delayMatch193/1 -> Accumulator_instance96/3(edge)
  delayMatch194/1 -> Accumulator_instance97/1(mode)
  delayMatch195/1 -> Accumulator_instance97/3(edge)
  delayMatch196/1 -> Accumulator_instance98/1(mode)
  delayMatch197/1 -> Accumulator_instance98/3(edge)
  delayMatch198/1 -> Accumulator_instance99/1(mode)
  delayMatch199/1 -> Accumulator_instance99/3(edge)
  delayMatch200/1 -> Accumulator_instance100/1(mode)
  delayMatch201/1 -> Accumulator_instance100/3(edge)
  delayMatch202/1 -> Accumulator_instance101/1(mode)
  delayMatch203/1 -> Accumulator_instance101/3(edge)
  delayMatch204/1 -> Accumulator_instance102/1(mode)
  delayMatch205/1 -> Accumulator_instance102/3(edge)
  delayMatch206/1 -> Accumulator_instance103/1(mode)
  delayMatch207/1 -> Accumulator_instance103/3(edge)
  delayMatch208/1 -> Accumulator_instance104/1(mode)
  delayMatch209/1 -> Accumulator_instance104/3(edge)
  delayMatch210/1 -> Accumulator_instance105/1(mode)
  delayMatch211/1 -> Accumulator_instance105/3(edge)
  delayMatch212/1 -> Accumulator_instance106/1(mode)
  delayMatch213/1 -> Accumulator_instance106/3(edge)
  delayMatch214/1 -> Accumulator_instance107/1(mode)
  delayMatch215/1 -> Accumulator_instance107/3(edge)
  delayMatch216/1 -> Accumulator_instance108/1(mode)
  delayMatch217/1 -> Accumulator_instance108/3(edge)
  delayMatch218/1 -> Accumulator_instance109/1(mode)
  delayMatch219/1 -> Accumulator_instance109/3(edge)
  delayMatch220/1 -> Accumulator_instance110/1(mode)
  delayMatch221/1 -> Accumulator_instance110/3(edge)
  delayMatch222/1 -> Accumulator_instance111/1(mode)
  delayMatch223/1 -> Accumulator_instance111/3(edge)
  delayMatch224/1 -> Accumulator_instance112/1(mode)
  delayMatch225/1 -> Accumulator_instance112/3(edge)
  delayMatch226/1 -> Accumulator_instance113/1(mode)
  delayMatch227/1 -> Accumulator_instance113/3(edge)
  delayMatch228/1 -> Accumulator_instance114/1(mode)
  delayMatch229/1 -> Accumulator_instance114/3(edge)
  delayMatch230/1 -> Accumulator_instance115/1(mode)
  delayMatch231/1 -> Accumulator_instance115/3(edge)
  delayMatch232/1 -> Accumulator_instance116/1(mode)
  delayMatch233/1 -> Accumulator_instance116/3(edge)
  delayMatch234/1 -> Accumulator_instance117/1(mode)
  delayMatch235/1 -> Accumulator_instance117/3(edge)
  delayMatch236/1 -> Accumulator_instance118/1(mode)
  delayMatch237/1 -> Accumulator_instance118/3(edge)
  delayMatch238/1 -> Accumulator_instance119/1(mode)
  delayMatch239/1 -> Accumulator_instance119/3(edge)
  delayMatch240/1 -> Accumulator_instance120/1(mode)
  delayMatch241/1 -> Accumulator_instance120/3(edge)
  delayMatch242/1 -> Accumulator_instance121/1(mode)
  delayMatch243/1 -> Accumulator_instance121/3(edge)
  delayMatch244/1 -> Accumulator_instance122/1(mode)
  delayMatch245/1 -> Accumulator_instance122/3(edge)
  delayMatch246/1 -> Accumulator_instance123/1(mode)
  delayMatch247/1 -> Accumulator_instance123/3(edge)
  delayMatch248/1 -> Accumulator_instance124/1(mode)
  delayMatch249/1 -> Accumulator_instance124/3(edge)
  delayMatch250/1 -> Accumulator_instance125/1(mode)
  delayMatch251/1 -> Accumulator_instance125/3(edge)
  delayMatch252/1 -> Accumulator_instance126/1(mode)
  delayMatch253/1 -> Accumulator_instance126/3(edge)
  delayMatch254/1 -> Accumulator_instance127/1(mode)
  delayMatch255/1 -> Accumulator_instance127/3(edge)
  delayMatch256/1 -> Accumulator_instance128/1(mode)
  delayMatch257/1 -> Accumulator_instance128/3(edge)
  delayMatch258/1 -> Accumulator_instance129/1(mode)
  delayMatch259/1 -> Accumulator_instance129/3(edge)
  delayMatch260/1 -> Accumulator_instance130/1(mode)
  delayMatch261/1 -> Accumulator_instance130/3(edge)
  delayMatch262/1 -> Accumulator_instance131/1(mode)
  delayMatch263/1 -> Accumulator_instance131/3(edge)
  delayMatch264/1 -> Accumulator_instance132/1(mode)
  delayMatch265/1 -> Accumulator_instance132/3(edge)
  delayMatch266/1 -> Accumulator_instance133/1(mode)
  delayMatch267/1 -> Accumulator_instance133/3(edge)
  delayMatch268/1 -> Accumulator_instance134/1(mode)
  delayMatch269/1 -> Accumulator_instance134/3(edge)
  delayMatch270/1 -> Accumulator_instance135/1(mode)
  delayMatch271/1 -> Accumulator_instance135/3(edge)
  delayMatch272/1 -> Accumulator_instance136/1(mode)
  delayMatch273/1 -> Accumulator_instance136/3(edge)
  delayMatch274/1 -> Accumulator_instance137/1(mode)
  delayMatch275/1 -> Accumulator_instance137/3(edge)
  delayMatch276/1 -> Accumulator_instance138/1(mode)
  delayMatch277/1 -> Accumulator_instance138/3(edge)
  delayMatch278/1 -> Accumulator_instance139/1(mode)
  delayMatch279/1 -> Accumulator_instance139/3(edge)
  delayMatch280/1 -> Accumulator_instance140/1(mode)
  delayMatch281/1 -> Accumulator_instance140/3(edge)
  delayMatch282/1 -> Accumulator_instance141/1(mode)
  delayMatch283/1 -> Accumulator_instance141/3(edge)
  delayMatch284/1 -> Accumulator_instance142/1(mode)
  delayMatch285/1 -> Accumulator_instance142/3(edge)
  delayMatch286/1 -> Accumulator_instance143/1(mode)
  delayMatch287/1 -> Accumulator_instance143/3(edge)
  delayMatch288/1 -> Accumulator_instance144/1(mode)
  delayMatch289/1 -> Accumulator_instance144/3(edge)
  delayMatch290/1 -> Accumulator_instance145/1(mode)
  delayMatch291/1 -> Accumulator_instance145/3(edge)
  delayMatch292/1 -> Accumulator_instance146/1(mode)
  delayMatch293/1 -> Accumulator_instance146/3(edge)
  delayMatch294/1 -> Accumulator_instance147/1(mode)
  delayMatch295/1 -> Accumulator_instance147/3(edge)
  delayMatch296/1 -> Accumulator_instance148/1(mode)
  delayMatch297/1 -> Accumulator_instance148/3(edge)
  delayMatch298/1 -> Accumulator_instance149/1(mode)
  delayMatch299/1 -> Accumulator_instance149/3(edge)
  delayMatch300/1 -> Accumulator_instance150/1(mode)
  delayMatch301/1 -> Accumulator_instance150/3(edge)
  delayMatch302/1 -> Accumulator_instance151/1(mode)
  delayMatch303/1 -> Accumulator_instance151/3(edge)
  delayMatch304/1 -> Accumulator_instance152/1(mode)
  delayMatch305/1 -> Accumulator_instance152/3(edge)
  delayMatch306/1 -> Accumulator_instance153/1(mode)
  delayMatch307/1 -> Accumulator_instance153/3(edge)
  delayMatch308/1 -> Accumulator_instance154/1(mode)
  delayMatch309/1 -> Accumulator_instance154/3(edge)
  delayMatch310/1 -> Accumulator_instance155/1(mode)
  delayMatch311/1 -> Accumulator_instance155/3(edge)
  delayMatch312/1 -> Accumulator_instance156/1(mode)
  delayMatch313/1 -> Accumulator_instance156/3(edge)
  delayMatch314/1 -> Accumulator_instance157/1(mode)
  delayMatch315/1 -> Accumulator_instance157/3(edge)
  delayMatch316/1 -> Accumulator_instance158/1(mode)
  delayMatch317/1 -> Accumulator_instance158/3(edge)
  delayMatch318/1 -> Accumulator_instance159/1(mode)
  delayMatch319/1 -> Accumulator_instance159/3(edge)
  delayMatch320/1 -> Accumulator_instance160/1(mode)
  delayMatch321/1 -> Accumulator_instance160/3(edge)
  delayMatch322/1 -> Accumulator_instance161/1(mode)
  delayMatch323/1 -> Accumulator_instance161/3(edge)
  delayMatch324/1 -> Accumulator_instance162/1(mode)
  delayMatch325/1 -> Accumulator_instance162/3(edge)
  delayMatch326/1 -> Accumulator_instance163/1(mode)
  delayMatch327/1 -> Accumulator_instance163/3(edge)
  delayMatch328/1 -> Accumulator_instance164/1(mode)
  delayMatch329/1 -> Accumulator_instance164/3(edge)
  delayMatch330/1 -> Accumulator_instance165/1(mode)
  delayMatch331/1 -> Accumulator_instance165/3(edge)
  delayMatch332/1 -> Accumulator_instance166/1(mode)
  delayMatch333/1 -> Accumulator_instance166/3(edge)
  delayMatch334/1 -> Accumulator_instance167/1(mode)
  delayMatch335/1 -> Accumulator_instance167/3(edge)
  delayMatch336/1 -> Accumulator_instance168/1(mode)
  delayMatch337/1 -> Accumulator_instance168/3(edge)
  delayMatch338/1 -> Accumulator_instance169/1(mode)
  delayMatch339/1 -> Accumulator_instance169/3(edge)
  delayMatch340/1 -> Accumulator_instance170/1(mode)
  delayMatch341/1 -> Accumulator_instance170/3(edge)
  delayMatch342/1 -> Accumulator_instance171/1(mode)
  delayMatch343/1 -> Accumulator_instance171/3(edge)
  delayMatch344/1 -> Accumulator_instance172/1(mode)
  delayMatch345/1 -> Accumulator_instance172/3(edge)
  delayMatch346/1 -> Accumulator_instance173/1(mode)
  delayMatch347/1 -> Accumulator_instance173/3(edge)
  delayMatch348/1 -> Accumulator_instance174/1(mode)
  delayMatch349/1 -> Accumulator_instance174/3(edge)
  delayMatch350/1 -> Accumulator_instance175/1(mode)
  delayMatch351/1 -> Accumulator_instance175/3(edge)
  delayMatch352/1 -> Accumulator_instance176/1(mode)
  delayMatch353/1 -> Accumulator_instance176/3(edge)
  delayMatch354/1 -> Accumulator_instance177/1(mode)
  delayMatch355/1 -> Accumulator_instance177/3(edge)
  delayMatch356/1 -> Accumulator_instance178/1(mode)
  delayMatch357/1 -> Accumulator_instance178/3(edge)
  delayMatch358/1 -> Accumulator_instance179/1(mode)
  delayMatch359/1 -> Accumulator_instance179/3(edge)
  delayMatch360/1 -> Accumulator_instance180/1(mode)
  delayMatch361/1 -> Accumulator_instance180/3(edge)
  Multiport Switch1/1 -> delayMatch361/1, delayMatch359/1, delayMatch357/1, delayMatch355/1, delayMatch353/1, delayMatch351/1, delayMatch349/1, delayMatch347/1, delayMatch345/1, delayMatch343/1, delayMatch341/1, delayMatch339/1, delayMatch337/1, delayMatch335/1, delayMatch333/1, delayMatch331/1, delayMatch329/1, delayMatch327/1, delayMatch325/1, delayMatch323/1, delayMatch321/1, delayMatch319/1, delayMatch317/1, delayMatch315/1, delayMatch313/1, delayMatch311/1, delayMatch309/1, delayMatch307/1, delayMatch305/1, delayMatch303/1, delayMatch301/1, delayMatch299/1, delayMatch297/1, delayMatch295/1, delayMatch293/1, delayMatch291/1, delayMatch289/1, delayMatch287/1, delayMatch285/1, delayMatch283/1, delayMatch281/1, delayMatch279/1, delayMatch277/1, delayMatch275/1, delayMatch273/1, delayMatch271/1, delayMatch269/1, delayMatch267/1, delayMatch265/1, delayMatch263/1, delayMatch261/1, delayMatch259/1, delayMatch257/1, delayMatch255/1, delayMatch253/1, delayMatch251/1, delayMatch249/1, delayMatch247/1, delayMatch245/1, delayMatch243/1, delayMatch241/1, delayMatch239/1, delayMatch237/1, delayMatch235/1, delayMatch233/1, delayMatch231/1, delayMatch229/1, delayMatch227/1, delayMatch225/1, delayMatch223/1, delayMatch221/1, delayMatch219/1, delayMatch217/1, delayMatch215/1, delayMatch213/1, delayMatch211/1, delayMatch209/1, delayMatch207/1, delayMatch205/1, delayMatch203/1, delayMatch201/1, delayMatch199/1, delayMatch197/1, delayMatch195/1, delayMatch193/1, delayMatch191/1, delayMatch189/1, delayMatch187/1, delayMatch185/1, delayMatch183/1, delayMatch181/1, delayMatch179/1, delayMatch177/1, delayMatch175/1, delayMatch173/1, delayMatch171/1, delayMatch169/1, delayMatch167/1, delayMatch165/1, delayMatch163/1, delayMatch161/1, delayMatch159/1, delayMatch157/1, delayMatch155/1, delayMatch153/1, delayMatch151/1, delayMatch149/1, delayMatch147/1, delayMatch145/1, delayMatch143/1, delayMatch141/1, delayMatch139/1, delayMatch137/1, delayMatch135/1, delayMatch133/1, delayMatch131/1, delayMatch129/1, delayMatch127/1, delayMatch125/1, delayMatch123/1, delayMatch121/1, delayMatch119/1, delayMatch117/1, delayMatch115/1, delayMatch113/1, delayMatch111/1, delayMatch109/1, delayMatch107/1, delayMatch105/1, delayMatch103/1, delayMatch101/1, delayMatch99/1, delayMatch97/1, delayMatch95/1, delayMatch93/1, delayMatch91/1, delayMatch89/1, delayMatch87/1, delayMatch85/1, delayMatch83/1, delayMatch81/1, delayMatch79/1, delayMatch77/1, delayMatch75/1, delayMatch73/1, delayMatch71/1, delayMatch69/1, delayMatch67/1, delayMatch65/1, delayMatch63/1, delayMatch61/1, delayMatch59/1, delayMatch57/1, delayMatch55/1, delayMatch53/1, delayMatch51/1, delayMatch49/1, delayMatch47/1, delayMatch45/1, delayMatch43/1, delayMatch41/1, delayMatch39/1, delayMatch37/1, delayMatch35/1, delayMatch33/1, delayMatch31/1, delayMatch29/1, delayMatch27/1, delayMatch25/1, delayMatch23/1, delayMatch21/1, delayMatch19/1, delayMatch17/1, delayMatch15/1, delayMatch13/1, delayMatch11/1, delayMatch9/1, delayMatch7/1, delayMatch5/1, delayMatch3/1
  Delay/1 -> delayMatch362/1
